simulink model "naikist"  (R2019a)
settings: Solver=VariableStepAuto  StartTime=0.0  StopTime=10.0  RelTol=1e-3
settings Model: Creator=toshi  LastModifiedBy=toshi

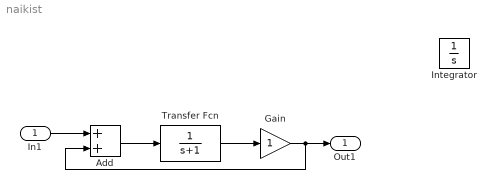
== system naikist ==
  In1 : Inport
  Add : Sum
  Gain : Gain
  Integrator : Integrator
  Transfer Fcn : TransferFcn  Denominator=[1 1]
  Out1 : Outport
  wires:
  Transfer Fcn/1 -> Gain/1
  In1/1 -> Add/1
  Add/1 -> Transfer Fcn/1
  Gain/1 -> Out1/1, Add/2
